simulink model "Lab6"  (R2016b)
settings: Solver=VariableStepAuto  StartTime=0.0  StopTime=1  RelTol=1e-3
libraries: dsparch4 x1
settings Model: Creator=mahbu  LastModifiedBy=mahbu

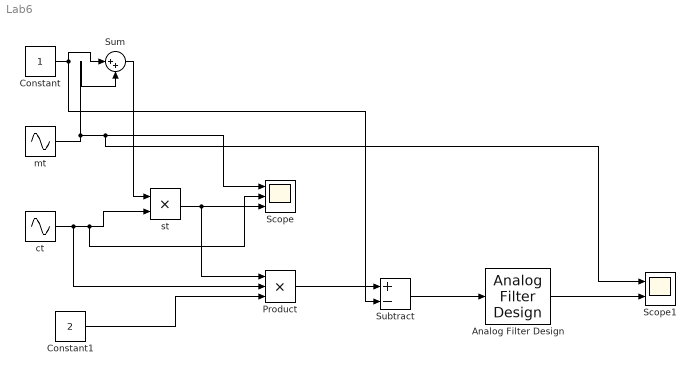
== system Lab6 ==
  Analog Filter Design : dsparch4/Analog Filter Design  method=Butterworth  filttype=Lowpass  N=8  Wlo=2*pi*7  Whi=80  Rp=2  Rs=40
  Constant : Constant
  Constant1 : Constant  Value=2
  Product : Product  Inputs=3
  Scope : Scope  NumInputPorts=3
  Scope1 : Scope  NumInputPorts=2
  Subtract : Sum  Inputs=+-
  Sum : Sum  Inputs=|++
  ct : Sin  Frequency=2*pi*100  Phase=pi/2  SampleTime=1/10000
  "mt " : Sin  Amplitude=2  Frequency=2*pi*5  SampleTime=1/10000
  st : Product
  wires:
  ct/1 -> Product/2, Scope/2, st/2
  Constant/1 -> Subtract/2, Sum/1
  Sum/1 -> st/1
  st/1 -> Product/1, Scope/3
  Constant1/1 -> Product/3
  Product/1 -> Subtract/1
  Subtract/1 -> Analog Filter Design/1
  Analog Filter Design/1 -> Scope1/2
  "mt "/1 -> Scope1/1, Scope/1, Sum/2
